simulink model "GoToTest"  (R2015b)
settings: Solver=VariableStepAuto  StartTime=0.0  StopTime=inf  RelTol=1e-3
libraries: aerolibanimutils x1, simulink x1, dspnetwork x1
(part 1 of 2)
settings Model: Creator=Ryuu  LastModifiedBy=Ryuu

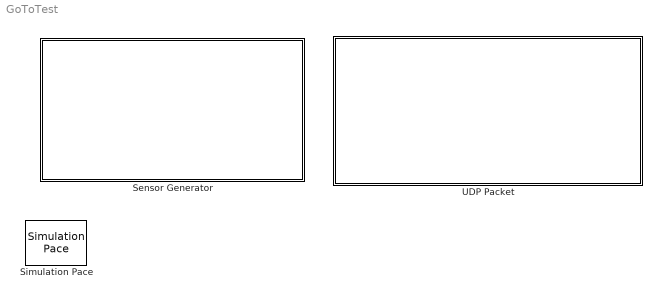
== system GoToTest ==
  "Sensor Generator " : Subsystem
  Simulation Pace : aerolibanimutils/Simulation Pace  SimulationPace=1  SleepMode=MATLAB Thread  OutputPaceError=off  SampleTime=1/30
  UDP Packet : Subsystem

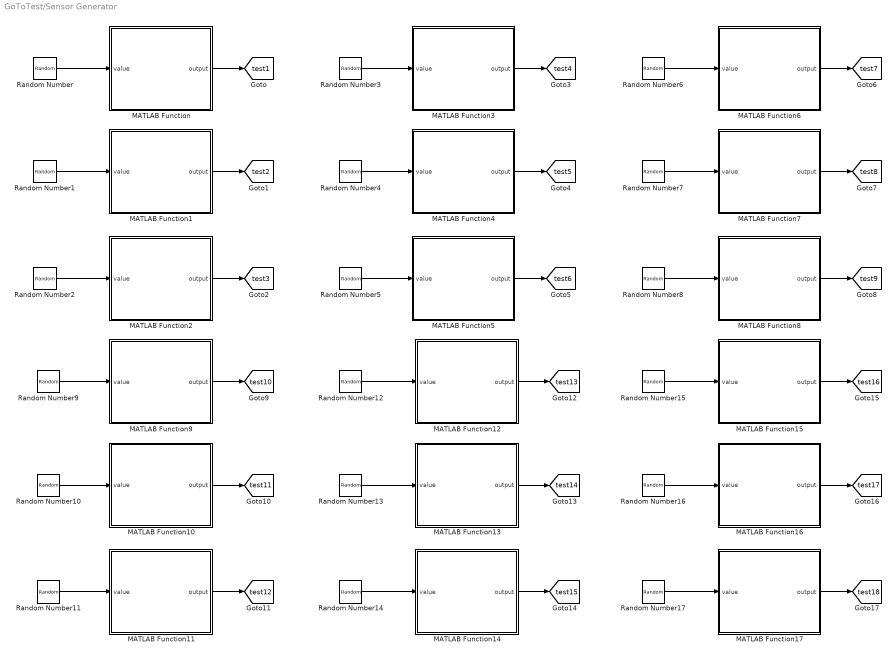
== system GoToTest/Sensor Generator  ==
  MATLAB Function : MATLAB Function  TreatAsAtomicUnit=on
  MATLAB Function1 : MATLAB Function  TreatAsAtomicUnit=on
  MATLAB Function10 : MATLAB Function  TreatAsAtomicUnit=on
  MATLAB Function11 : MATLAB Function  TreatAsAtomicUnit=on
  MATLAB Function12 : MATLAB Function  TreatAsAtomicUnit=on
  MATLAB Function13 : MATLAB Function  TreatAsAtomicUnit=on
  MATLAB Function14 : MATLAB Function  TreatAsAtomicUnit=on
  MATLAB Function15 : MATLAB Function  TreatAsAtomicUnit=on
  MATLAB Function16 : MATLAB Function  TreatAsAtomicUnit=on
  MATLAB Function17 : MATLAB Function  TreatAsAtomicUnit=on
  MATLAB Function2 : MATLAB Function  TreatAsAtomicUnit=on
  MATLAB Function3 : MATLAB Function  TreatAsAtomicUnit=on
  MATLAB Function4 : MATLAB Function  TreatAsAtomicUnit=on
  MATLAB Function5 : MATLAB Function  TreatAsAtomicUnit=on
  MATLAB Function6 : MATLAB Function  TreatAsAtomicUnit=on
  MATLAB Function7 : MATLAB Function  TreatAsAtomicUnit=on
  MATLAB Function8 : MATLAB Function  TreatAsAtomicUnit=on
  MATLAB Function9 : MATLAB Function  TreatAsAtomicUnit=on
  Random Number : RandomNumber  Mean=100  Variance=50  Seed=1  SampleTime=0.02
  Random Number1 : RandomNumber  Mean=100  Variance=50  Seed=2  SampleTime=0.02
  Random Number10 : RandomNumber  Mean=100  Variance=50  Seed=11  SampleTime=0.02
  Random Number11 : RandomNumber  Mean=100  Variance=50  Seed=12  SampleTime=0.02
  Random Number12 : RandomNumber  Mean=100  Variance=50  Seed=13  SampleTime=0.02
  Random Number13 : RandomNumber  Mean=100  Variance=50  Seed=14  SampleTime=0.02
  Random Number14 : RandomNumber  Mean=100  Variance=50  Seed=15  SampleTime=0.02
  Random Number15 : RandomNumber  Mean=100  Variance=50  Seed=16  SampleTime=0.02
  Random Number16 : RandomNumber  Mean=100  Variance=50  Seed=17  SampleTime=0.02
  Random Number17 : RandomNumber  Mean=100  Variance=50  Seed=18  SampleTime=0.02
  Random Number2 : RandomNumber  Mean=100  Variance=50  Seed=3  SampleTime=0.02
  Random Number3 : RandomNumber  Mean=100  Variance=50  Seed=4  SampleTime=0.02
  Random Number4 : RandomNumber  Mean=100  Variance=50  Seed=5  SampleTime=0.02
  Random Number5 : RandomNumber  Mean=100  Variance=50  Seed=6  SampleTime=0.02
  Random Number6 : RandomNumber  Mean=100  Variance=50  Seed=7  SampleTime=0.02
  Random Number7 : RandomNumber  Mean=100  Variance=50  Seed=8  SampleTime=0.02
  Random Number8 : RandomNumber  Mean=100  Variance=50  Seed=9  SampleTime=0.02
  Random Number9 : RandomNumber  Mean=100  Variance=50  Seed=10  SampleTime=0.02
  tag scope: test10=global, test11=global, test12=global, test13=global, test14=global, test15=global, test16=global, test17=global, test18=global, test1=global, test2=global, test3=global, test4=global, test5=global, test6=global, test7=global, test8=global, test9=global
  wires:
  Random Number/1 -> MATLAB Function/1(value)
  MATLAB Function/1(output) -> [test1]
  Random Number1/1 -> MATLAB Function1/1(value)
  MATLAB Function1/1(output) -> [test2]
  Random Number2/1 -> MATLAB Function2/1(value)
  MATLAB Function2/1(output) -> [test3]
  Random Number3/1 -> MATLAB Function3/1(value)
  MATLAB Function3/1(output) -> [test4]
  Random Number4/1 -> MATLAB Function4/1(value)
  MATLAB Function4/1(output) -> [test5]
  Random Number5/1 -> MATLAB Function5/1(value)
  MATLAB Function5/1(output) -> [test6]
  Random Number6/1 -> MATLAB Function6/1(value)
  MATLAB Function6/1(output) -> [test7]
  Random Number7/1 -> MATLAB Function7/1(value)
  MATLAB Function7/1(output) -> [test8]
  Random Number8/1 -> MATLAB Function8/1(value)
  MATLAB Function8/1(output) -> [test9]
  Random Number9/1 -> MATLAB Function9/1(value)
  MATLAB Function9/1(output) -> [test10]
  Random Number10/1 -> MATLAB Function10/1(value)
  MATLAB Function10/1(output) -> [test11]
  Random Number11/1 -> MATLAB Function11/1(value)
  MATLAB Function11/1(output) -> [test12]
  Random Number12/1 -> MATLAB Function12/1(value)
  MATLAB Function12/1(output) -> [test13]
  Random Number13/1 -> MATLAB Function13/1(value)
  MATLAB Function13/1(output) -> [test14]
  Random Number14/1 -> MATLAB Function14/1(value)
  MATLAB Function14/1(output) -> [test15]
  Random Number15/1 -> MATLAB Function15/1(value)
  MATLAB Function15/1(output) -> [test16]
  Random Number16/1 -> MATLAB Function16/1(value)
  MATLAB Function16/1(output) -> [test17]
  Random Number17/1 -> MATLAB Function17/1(value)
  MATLAB Function17/1(output) -> [test18]

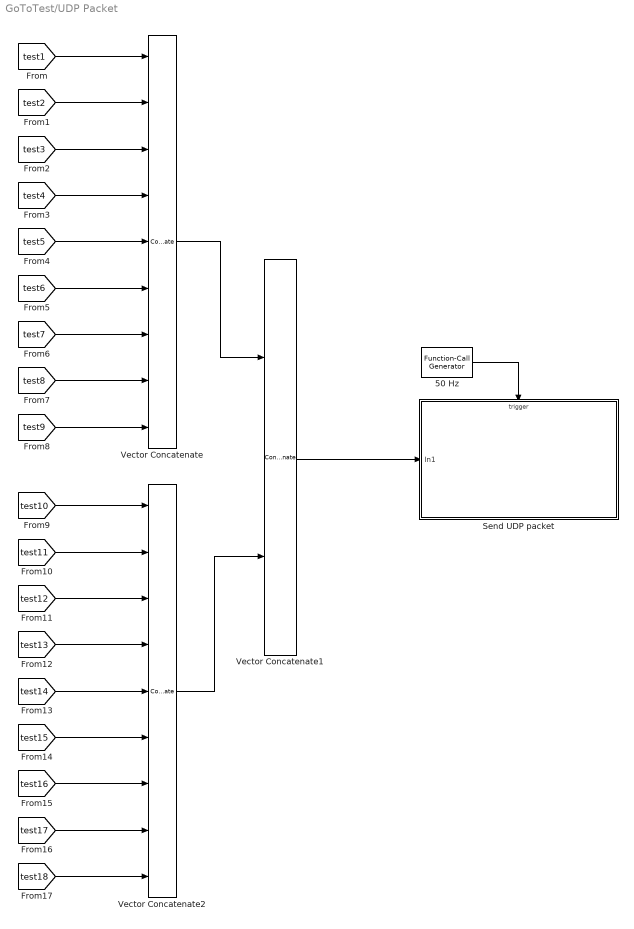
== system GoToTest/UDP Packet ==
  50 Hz : simulink/Ports & Subsystems/Function-Call Generator  sample_time=0.02  numberOfIterations=1
  Send UDP packet : Subsystem
  Vector Concatenate : Concatenate  NumInputs=9
  Vector Concatenate1 : Concatenate
  Vector Concatenate2 : Concatenate  NumInputs=9
  wires:
  [test1] -> Vector Concatenate/1
  50 Hz/1 -> Send UDP packet/Trigger
  Vector Concatenate/1 -> Vector Concatenate1/1
  [test2] -> Vector Concatenate/2
  [test3] -> Vector Concatenate/3
  [test4] -> Vector Concatenate/4
  [test5] -> Vector Concatenate/5
  [test6] -> Vector Concatenate/6
  [test7] -> Vector Concatenate/7
  [test8] -> Vector Concatenate/8
  [test9] -> Vector Concatenate/9
  [test10] -> Vector Concatenate2/1
  [test11] -> Vector Concatenate2/2
  [test12] -> Vector Concatenate2/3
  [test13] -> Vector Concatenate2/4
  [test14] -> Vector Concatenate2/5
  [test15] -> Vector Concatenate2/6
  [test16] -> Vector Concatenate2/7
  [test17] -> Vector Concatenate2/8
  [test18] -> Vector Concatenate2/9
  Vector Concatenate2/1 -> Vector Concatenate1/2
  Vector Concatenate1/1 -> Send UDP packet/1(In1)

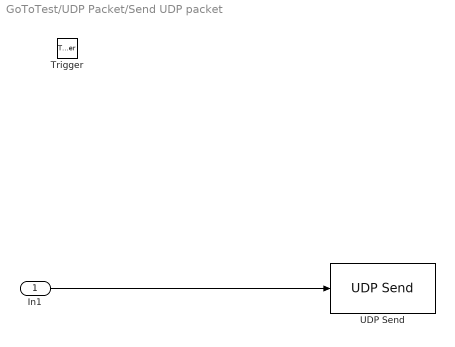
== system GoToTest/UDP Packet/Send UDP packet ==
  In1 : Inport
  Trigger : TriggerPort  TriggerType=function-call  PortDimensions=1
  UDP Send : dspnetwork/UDP Send  remoteURL='192.168.21.1'  remotePort=25000  localURL='0.0.0.0'  localPortSource=Automatically determine  localPort=-1  sampletime=-1  separateLengthPort=0
  wires:
  In1/1 -> UDP Send/1

== matlab function GoToTest/Sensor Generator /MATLAB Function1 ==
  data: value input; output output uint8 size=1000
function output = data_serialize(value)
label = 'Test 2';
type = 'Testsensor 2';
min = 24;
max = 45;

label_ser = sensor_serialize(label);
type_ser = sensor_serialize(type);
value_ser = sensor_serialize(value);
min_ser = sensor_serialize(min);
max_ser = sensor_serialize(max);


V = length(label_ser);
W = length(type_ser);
X = length(value_ser);
Y = length(min_ser);
Z = length(max_ser);

output = [
    label_ser;
    type_ser;
    value_ser;
    min_ser;
    max_ser;
    ];
end


function m = sensor_serialize(v)
    % dispatch according to type
    if isnumeric(v) 
        m = serialize_numeric(v);
    elseif ischar(v)
        m = serialize_string(v);
    elseif islogical(v)
        m = serialize_logical(v);
	else
		error('Unsupported data type');
    end
end

% single scalar
function m = serialize_scalar(v)
    % Data type & data
    m = [class2tag(class(v)); typecast(v,'uint8').'];
end

% char arrays
function m = serialize_string(v)
    if size(v,1) == 1
        % horizontal string: Type, Length, and Data
        m = [uint8(0); typecast(uint32(length(v)),'uint8').'; uint8(v(:))];
    elseif sum(size(v)) == 0
        % '': special encoding
        m = uint8(200);
    else
        % general char array: Tag & Number of dimensions, Dimensions, Data
        m = [uint8(132); ndims(v); typecast(uint32(size(v)),'uint8').'; uint8(v(:))];
    end
end

% logical arrays
function m = serialize_logical(v)
    % Tag & Number of dimensions, Dimensions, Data
    m = [uint8(133); ndims(v); typecast(uint32(size(v)),'uint8').'; uint8(v(:))];
end

% non-complex and non-sparse numerical matrix
function m = serialize_numeric_simple(v)
    % Tag & Number of dimensions, Dimensions, Data
    m = [16+class2tag(class(v)); ndims(v); typecast(uint32(size(v)),'uint8').'; typecast(v(:).','uint8').'];
end

% Numeric Matrix: can be real/complex, sparse/full, scalar
function m = serialize_numeric(v)
    if issparse(v)
        % Data Type & Dimensions
        m = [uint8(130); typecast(uint64(size(v,1)), 'uint8').'; typecast(uint64(size(v,2)), 'uint8').']; % vectorize
        % Index vectors
        [i,j,s] = find(v);        
        % Real/Complex
        if isreal(v)
            m = [m; serialize_numeric_simple(i); serialize_numeric_simple(j); 1; serialize_numeric_simple(s)];
        else
            m = [m; serialize_numeric_simple(i); serialize_numeric_simple(j); 0; serialize_numeric_simple(real(s)); serialize_numeric_simple(imag(s))];
        end
    elseif ~isreal(v)
        % Data type & contents
        m = [uint8(131); serialize_numeric_simple(real(v)); serialize_numeric_simple(imag(v))];
    elseif isscalar(v)
        % Scalar
        m = serialize_scalar(v);
    else
        % Simple matrix
        m = serialize_numeric_simple(v);
    end
end

% *container* class to byte
function b = class2tag(cls)
	switch cls
		case 'string'
            b = uint8(0);
		case 'double'
			b = uint8(1);
		case 'single'
			b = uint8(2);
		case 'int8'
			b = uint8(3);
		case 'uint8'
			b = uint8(4);
		case 'int16'
			b = uint8(5);
		case 'uint16'
			b = uint8(6);
		case 'int32'
			b = uint8(7);
		case 'uint32'
			b = uint8(8);
		case 'int64'
			b = uint8(9);
		case 'uint64'
			b = uint8(10);
		otherwise
			error('Unknown class');
    end
end

== matlab function GoToTest/Sensor Generator /MATLAB Function ==
  data: value input; output output uint8 size=1000
function output = data_serialize(value)
label = 'Test 1';
type = 'Testsensor 1';
min = 24;
max = 45;

label_ser = sensor_serialize(label);
type_ser = sensor_serialize(type);
value_ser = sensor_serialize(value);
min_ser = sensor_serialize(min);
max_ser = sensor_serialize(max);


V = length(label_ser);
W = length(type_ser);
X = length(value_ser);
Y = length(min_ser);
Z = length(max_ser);

output = [
    label_ser;
    type_ser;
    value_ser;
    min_ser;
    max_ser;
    ];
end


function m = sensor_serialize(v)
    % dispatch according to type
    if isnumeric(v) 
        m = serialize_numeric(v);
    elseif ischar(v)
        m = serialize_string(v);
    elseif islogical(v)
        m = serialize_logical(v);
	else
		error('Unsupported data type');
    end
end

% single scalar
function m = serialize_scalar(v)
    % Data type & data
    m = [class2tag(class(v)); typecast(v,'uint8').'];
end

% char arrays
function m = serialize_string(v)
    if size(v,1) == 1
        % horizontal string: Type, Length, and Data
        m = [uint8(0); typecast(uint32(length(v)),'uint8').'; uint8(v(:))];
    elseif sum(size(v)) == 0
        % '': special encoding
        m = uint8(200);
    else
        % general char array: Tag & Number of dimensions, Dimensions, Data
        m = [uint8(132); ndims(v); typecast(uint32(size(v)),'uint8').'; uint8(v(:))];
    end
end

% logical arrays
function m = serialize_logical(v)
    % Tag & Number of dimensions, Dimensions, Data
    m = [uint8(133); ndims(v); typecast(uint32(size(v)),'uint8').'; uint8(v(:))];
end

% non-complex and non-sparse numerical matrix
function m = serialize_numeric_simple(v)
    % Tag & Number of dimensions, Dimensions, Data
    m = [16+class2tag(class(v)); ndims(v); typecast(uint32(size(v)),'uint8').'; typecast(v(:).','uint8').'];
end

% Numeric Matrix: can be real/complex, sparse/full, scalar
function m = serialize_numeric(v)
    if issparse(v)
        % Data Type & Dimensions
        m = [uint8(130); typecast(uint64(size(v,1)), 'uint8').'; typecast(uint64(size(v,2)), 'uint8').']; % vectorize
        % Index vectors
        [i,j,s] = find(v);        
        % Real/Complex
        if isreal(v)
            m = [m; serialize_numeric_simple(i); serialize_numeric_simple(j); 1; serialize_numeric_simple(s)];
        else
            m = [m; serialize_numeric_simple(i); serialize_numeric_simple(j); 0; serialize_numeric_simple(real(s)); serialize_numeric_simple(imag(s))];
        end
    elseif ~isreal(v)
        % Data type & contents
        m = [uint8(131); serialize_numeric_simple(real(v)); serialize_numeric_simple(imag(v))];
    elseif isscalar(v)
        % Scalar
        m = serialize_scalar(v);
    else
        % Simple matrix
        m = serialize_numeric_simple(v);
    end
end

% *container* class to byte
function b = class2tag(cls)
	switch cls
		case 'string'
            b = uint8(0);
		case 'double'
			b = uint8(1);
		case 'single'
			b = uint8(2);
		case 'int8'
			b = uint8(3);
		case 'uint8'
			b = uint8(4);
		case 'int16'
			b = uint8(5);
		case 'uint16'
			b = uint8(6);
		case 'int32'
			b = uint8(7);
		case 'uint32'
			b = uint8(8);
		case 'int64'
			b = uint8(9);
		case 'uint64'
			b = uint8(10);
		otherwise
			error('Unknown class');
    end
end

== matlab function GoToTest/Sensor Generator /MATLAB Function2 ==
  data: value input; output output uint8 size=1000
function output = data_serialize(value)
label = 'Test 3';
type = 'Testsensor 3';
min = 24;
max = 45;

label_ser = sensor_serialize(label);
type_ser = sensor_serialize(type);
value_ser = sensor_serialize(value);
min_ser = sensor_serialize(min);
max_ser = sensor_serialize(max);


V = length(label_ser);
W = length(type_ser);
X = length(value_ser);
Y = length(min_ser);
Z = length(max_ser);

output = [
    label_ser;
    type_ser;
    value_ser;
    min_ser;
    max_ser;
    ];
end


function m = sensor_serialize(v)
    % dispatch according to type
    if isnumeric(v) 
        m = serialize_numeric(v);
    elseif ischar(v)
        m = serialize_string(v);
    elseif islogical(v)
        m = serialize_logical(v);
	else
		error('Unsupported data type');
    end
end

% single scalar
function m = serialize_scalar(v)
    % Data type & data
    m = [class2tag(class(v)); typecast(v,'uint8').'];
end

% char arrays
function m = serialize_string(v)
    if size(v,1) == 1
        % horizontal string: Type, Length, and Data
        m = [uint8(0); typecast(uint32(length(v)),'uint8').'; uint8(v(:))];
    elseif sum(size(v)) == 0
        % '': special encoding
        m = uint8(200);
    else
        % general char array: Tag & Number of dimensions, Dimensions, Data
        m = [uint8(132); ndims(v); typecast(uint32(size(v)),'uint8').'; uint8(v(:))];
    end
end

% logical arrays
function m = serialize_logical(v)
    % Tag & Number of dimensions, Dimensions, Data
    m = [uint8(133); ndims(v); typecast(uint32(size(v)),'uint8').'; uint8(v(:))];
end

% non-complex and non-sparse numerical matrix
function m = serialize_numeric_simple(v)
    % Tag & Number of dimensions, Dimensions, Data
    m = [16+class2tag(class(v)); ndims(v); typecast(uint32(size(v)),'uint8').'; typecast(v(:).','uint8').'];
end

% Numeric Matrix: can be real/complex, sparse/full, scalar
function m = serialize_numeric(v)
    if issparse(v)
        % Data Type & Dimensions
        m = [uint8(130); typecast(uint64(size(v,1)), 'uint8').'; typecast(uint64(size(v,2)), 'uint8').']; % vectorize
        % Index vectors
        [i,j,s] = find(v);        
        % Real/Complex
        if isreal(v)
            m = [m; serialize_numeric_simple(i); serialize_numeric_simple(j); 1; serialize_numeric_simple(s)];
        else
            m = [m; serialize_numeric_simple(i); serialize_numeric_simple(j); 0; serialize_numeric_simple(real(s)); serialize_numeric_simple(imag(s))];
        end
    elseif ~isreal(v)
        % Data type & contents
        m = [uint8(131); serialize_numeric_simple(real(v)); serialize_numeric_simple(imag(v))];
    elseif isscalar(v)
        % Scalar
        m = serialize_scalar(v);
    else
        % Simple matrix
        m = serialize_numeric_simple(v);
    end
end

% *container* class to byte
function b = class2tag(cls)
	switch cls
		case 'string'
            b = uint8(0);
		case 'double'
			b = uint8(1);
		case 'single'
			b = uint8(2);
		case 'int8'
			b = uint8(3);
		case 'uint8'
			b = uint8(4);
		case 'int16'
			b = uint8(5);
		case 'uint16'
			b = uint8(6);
		case 'int32'
			b = uint8(7);
		case 'uint32'
			b = uint8(8);
		case 'int64'
			b = uint8(9);
		case 'uint64'
			b = uint8(10);
		otherwise
			error('Unknown class');
    end
end

== matlab function GoToTest/Sensor Generator /MATLAB Function3 ==
  data: value input; output output uint8 size=1000
function output = data_serialize(value)
label = 'Test 4';
type = 'Testsensor 4';
min = 24;
max = 45;

label_ser = sensor_serialize(label);
type_ser = sensor_serialize(type);
value_ser = sensor_serialize(value);
min_ser = sensor_serialize(min);
max_ser = sensor_serialize(max);


V = length(label_ser);
W = length(type_ser);
X = length(value_ser);
Y = length(min_ser);
Z = length(max_ser);

output = [
    label_ser;
    type_ser;
    value_ser;
    min_ser;
    max_ser;
    ];
end


function m = sensor_serialize(v)
    % dispatch according to type
    if isnumeric(v) 
        m = serialize_numeric(v);
    elseif ischar(v)
        m = serialize_string(v);
    elseif islogical(v)
        m = serialize_logical(v);
	else
		error('Unsupported data type');
    end
end

% single scalar
function m = serialize_scalar(v)
    % Data type & data
    m = [class2tag(class(v)); typecast(v,'uint8').'];
end

% char arrays
function m = serialize_string(v)
    if size(v,1) == 1
        % horizontal string: Type, Length, and Data
        m = [uint8(0); typecast(uint32(length(v)),'uint8').'; uint8(v(:))];
    elseif sum(size(v)) == 0
        % '': special encoding
        m = uint8(200);
    else
        % general char array: Tag & Number of dimensions, Dimensions, Data
        m = [uint8(132); ndims(v); typecast(uint32(size(v)),'uint8').'; uint8(v(:))];
    end
end

% logical arrays
function m = serialize_logical(v)
    % Tag & Number of dimensions, Dimensions, Data
    m = [uint8(133); ndims(v); typecast(uint32(size(v)),'uint8').'; uint8(v(:))];
end

% non-complex and non-sparse numerical matrix
function m = serialize_numeric_simple(v)
    % Tag & Number of dimensions, Dimensions, Data
    m = [16+class2tag(class(v)); ndims(v); typecast(uint32(size(v)),'uint8').'; typecast(v(:).','uint8').'];
end

% Numeric Matrix: can be real/complex, sparse/full, scalar
function m = serialize_numeric(v)
    if issparse(v)
        % Data Type & Dimensions
        m = [uint8(130); typecast(uint64(size(v,1)), 'uint8').'; typecast(uint64(size(v,2)), 'uint8').']; % vectorize
        % Index vectors
        [i,j,s] = find(v);        
        % Real/Complex
        if isreal(v)
            m = [m; serialize_numeric_simple(i); serialize_numeric_simple(j); 1; serialize_numeric_simple(s)];
        else
            m = [m; serialize_numeric_simple(i); serialize_numeric_simple(j); 0; serialize_numeric_simple(real(s)); serialize_numeric_simple(imag(s))];
        end
    elseif ~isreal(v)
        % Data type & contents
        m = [uint8(131); serialize_numeric_simple(real(v)); serialize_numeric_simple(imag(v))];
    elseif isscalar(v)
        % Scalar
        m = serialize_scalar(v);
    else
        % Simple matrix
        m = serialize_numeric_simple(v);
    end
end

% *container* class to byte
function b = class2tag(cls)
	switch cls
		case 'string'
            b = uint8(0);
		case 'double'
			b = uint8(1);
		case 'single'
			b = uint8(2);
		case 'int8'
			b = uint8(3);
		case 'uint8'
			b = uint8(4);
		case 'int16'
			b = uint8(5);
		case 'uint16'
			b = uint8(6);
		case 'int32'
			b = uint8(7);
		case 'uint32'
			b = uint8(8);
		case 'int64'
			b = uint8(9);
		case 'uint64'
			b = uint8(10);
		otherwise
			error('Unknown class');
    end
end

== matlab function GoToTest/Sensor Generator /MATLAB Function4 ==
  data: value input; output output uint8 size=1000
function output = data_serialize(value)
label = 'Test 5';
type = 'Testsensor 5';
min = 24;
max = 45;

label_ser = sensor_serialize(label);
type_ser = sensor_serialize(type);
value_ser = sensor_serialize(value);
min_ser = sensor_serialize(min);
max_ser = sensor_serialize(max);


V = length(label_ser);
W = length(type_ser);
X = length(value_ser);
Y = length(min_ser);
Z = length(max_ser);

output = [
    label_ser;
    type_ser;
    value_ser;
    min_ser;
    max_ser;
    ];
end


function m = sensor_serialize(v)
    % dispatch according to type
    if isnumeric(v) 
        m = serialize_numeric(v);
    elseif ischar(v)
        m = serialize_string(v);
    elseif islogical(v)
        m = serialize_logical(v);
	else
		error('Unsupported data type');
    end
end

% single scalar
function m = serialize_scalar(v)
    % Data type & data
    m = [class2tag(class(v)); typecast(v,'uint8').'];
end

% char arrays
function m = serialize_string(v)
    if size(v,1) == 1
        % horizontal string: Type, Length, and Data
        m = [uint8(0); typecast(uint32(length(v)),'uint8').'; uint8(v(:))];
    elseif sum(size(v)) == 0
        % '': special encoding
        m = uint8(200);
    else
        % general char array: Tag & Number of dimensions, Dimensions, Data
        m = [uint8(132); ndims(v); typecast(uint32(size(v)),'uint8').'; uint8(v(:))];
    end
end

% logical arrays
function m = serialize_logical(v)
    % Tag & Number of dimensions, Dimensions, Data
    m = [uint8(133); ndims(v); typecast(uint32(size(v)),'uint8').'; uint8(v(:))];
end

% non-complex and non-sparse numerical matrix
function m = serialize_numeric_simple(v)
    % Tag & Number of dimensions, Dimensions, Data
    m = [16+class2tag(class(v)); ndims(v); typecast(uint32(size(v)),'uint8').'; typecast(v(:).','uint8').'];
end

% Numeric Matrix: can be real/complex, sparse/full, scalar
function m = serialize_numeric(v)
    if issparse(v)
        % Data Type & Dimensions
        m = [uint8(130); typecast(uint64(size(v,1)), 'uint8').'; typecast(uint64(size(v,2)), 'uint8').']; % vectorize
        % Index vectors
        [i,j,s] = find(v);        
        % Real/Complex
        if isreal(v)
            m = [m; serialize_numeric_simple(i); serialize_numeric_simple(j); 1; serialize_numeric_simple(s)];
        else
            m = [m; serialize_numeric_simple(i); serialize_numeric_simple(j); 0; serialize_numeric_simple(real(s)); serialize_numeric_simple(imag(s))];
        end
    elseif ~isreal(v)
        % Data type & contents
        m = [uint8(131); serialize_numeric_simple(real(v)); serialize_numeric_simple(imag(v))];
    elseif isscalar(v)
        % Scalar
        m = serialize_scalar(v);
    else
        % Simple matrix
        m = serialize_numeric_simple(v);
    end
end

% *container* class to byte
function b = class2tag(cls)
	switch cls
		case 'string'
            b = uint8(0);
		case 'double'
			b = uint8(1);
		case 'single'
			b = uint8(2);
		case 'int8'
			b = uint8(3);
		case 'uint8'
			b = uint8(4);
		case 'int16'
			b = uint8(5);
		case 'uint16'
			b = uint8(6);
		case 'int32'
			b = uint8(7);
		case 'uint32'
			b = uint8(8);
		case 'int64'
			b = uint8(9);
		case 'uint64'
			b = uint8(10);
		otherwise
			error('Unknown class');
    end
end

== matlab function GoToTest/Sensor Generator /MATLAB Function5 ==
  data: value input; output output uint8 size=1000
function output = data_serialize(value)
label = 'Test 6';
type = 'Testsensor 6';
min = 24;
max = 45;

label_ser = sensor_serialize(label);
type_ser = sensor_serialize(type);
value_ser = sensor_serialize(value);
min_ser = sensor_serialize(min);
max_ser = sensor_serialize(max);


V = length(label_ser);
W = length(type_ser);
X = length(value_ser);
Y = length(min_ser);
Z = length(max_ser);

output = [
    label_ser;
    type_ser;
    value_ser;
    min_ser;
    max_ser;
    ];
end


function m = sensor_serialize(v)
    % dispatch according to type
    if isnumeric(v) 
        m = serialize_numeric(v);
    elseif ischar(v)
        m = serialize_string(v);
    elseif islogical(v)
        m = serialize_logical(v);
	else
		error('Unsupported data type');
    end
end

% single scalar
function m = serialize_scalar(v)
    % Data type & data
    m = [class2tag(class(v)); typecast(v,'uint8').'];
end

% char arrays
function m = serialize_string(v)
    if size(v,1) == 1
        % horizontal string: Type, Length, and Data
        m = [uint8(0); typecast(uint32(length(v)),'uint8').'; uint8(v(:))];
    elseif sum(size(v)) == 0
        % '': special encoding
        m = uint8(200);
    else
        % general char array: Tag & Number of dimensions, Dimensions, Data
        m = [uint8(132); ndims(v); typecast(uint32(size(v)),'uint8').'; uint8(v(:))];
    end
end

% logical arrays
function m = serialize_logical(v)
    % Tag & Number of dimensions, Dimensions, Data
    m = [uint8(133); ndims(v); typecast(uint32(size(v)),'uint8').'; uint8(v(:))];
end

% non-complex and non-sparse numerical matrix
function m = serialize_numeric_simple(v)
    % Tag & Number of dimensions, Dimensions, Data
    m = [16+class2tag(class(v)); ndims(v); typecast(uint32(size(v)),'uint8').'; typecast(v(:).','uint8').'];
end

% Numeric Matrix: can be real/complex, sparse/full, scalar
function m = serialize_numeric(v)
    if issparse(v)
        % Data Type & Dimensions
        m = [uint8(130); typecast(uint64(size(v,1)), 'uint8').'; typecast(uint64(size(v,2)), 'uint8').']; % vectorize
        % Index vectors
        [i,j,s] = find(v);        
        % Real/Complex
        if isreal(v)
            m = [m; serialize_numeric_simple(i); serialize_numeric_simple(j); 1; serialize_numeric_simple(s)];
        else
            m = [m; serialize_numeric_simple(i); serialize_numeric_simple(j); 0; serialize_numeric_simple(real(s)); serialize_numeric_simple(imag(s))];
        end
    elseif ~isreal(v)
        % Data type & contents
        m = [uint8(131); serialize_numeric_simple(real(v)); serialize_numeric_simple(imag(v))];
    elseif isscalar(v)
        % Scalar
        m = serialize_scalar(v);
    else
        % Simple matrix
        m = serialize_numeric_simple(v);
    end
end

% *container* class to byte
function b = class2tag(cls)
	switch cls
		case 'string'
            b = uint8(0);
		case 'double'
			b = uint8(1);
		case 'single'
			b = uint8(2);
		case 'int8'
			b = uint8(3);
		case 'uint8'
			b = uint8(4);
		case 'int16'
			b = uint8(5);
		case 'uint16'
			b = uint8(6);
		case 'int32'
			b = uint8(7);
		case 'uint32'
			b = uint8(8);
		case 'int64'
			b = uint8(9);
		case 'uint64'
			b = uint8(10);
		otherwise
			error('Unknown class');
    end
end

== matlab function GoToTest/Sensor Generator /MATLAB Function6 ==
  data: value input; output output uint8 size=1000
function output = data_serialize(value)
label = 'Test 7';
type = 'Testsensor 7';
min = 24;
max = 45;

label_ser = sensor_serialize(label);
type_ser = sensor_serialize(type);
value_ser = sensor_serialize(value);
min_ser = sensor_serialize(min);
max_ser = sensor_serialize(max);


V = length(label_ser);
W = length(type_ser);
X = length(value_ser);
Y = length(min_ser);
Z = length(max_ser);

output = [
    label_ser;
    type_ser;
    value_ser;
    min_ser;
    max_ser;
    ];
end


function m = sensor_serialize(v)
    % dispatch according to type
    if isnumeric(v) 
        m = serialize_numeric(v);
    elseif ischar(v)
        m = serialize_string(v);
    elseif islogical(v)
        m = serialize_logical(v);
	else
		error('Unsupported data type');
    end
end

% single scalar
function m = serialize_scalar(v)
    % Data type & data
    m = [class2tag(class(v)); typecast(v,'uint8').'];
end

% char arrays
function m = serialize_string(v)
    if size(v,1) == 1
        % horizontal string: Type, Length, and Data
        m = [uint8(0); typecast(uint32(length(v)),'uint8').'; uint8(v(:))];
    elseif sum(size(v)) == 0
        % '': special encoding
        m = uint8(200);
    else
        % general char array: Tag & Number of dimensions, Dimensions, Data
        m = [uint8(132); ndims(v); typecast(uint32(size(v)),'uint8').'; uint8(v(:))];
    end
end

% logical arrays
function m = serialize_logical(v)
    % Tag & Number of dimensions, Dimensions, Data
    m = [uint8(133); ndims(v); typecast(uint32(size(v)),'uint8').'; uint8(v(:))];
end

% non-complex and non-sparse numerical matrix
function m = serialize_numeric_simple(v)
    % Tag & Number of dimensions, Dimensions, Data
    m = [16+class2tag(class(v)); ndims(v); typecast(uint32(size(v)),'uint8').'; typecast(v(:).','uint8').'];
end

% Numeric Matrix: can be real/complex, sparse/full, scalar
function m = serialize_numeric(v)
    if issparse(v)
        % Data Type & Dimensions
        m = [uint8(130); typecast(uint64(size(v,1)), 'uint8').'; typecast(uint64(size(v,2)), 'uint8').']; % vectorize
        % Index vectors
        [i,j,s] = find(v);        
        % Real/Complex
        if isreal(v)
            m = [m; serialize_numeric_simple(i); serialize_numeric_simple(j); 1; serialize_numeric_simple(s)];
        else
            m = [m; serialize_numeric_simple(i); serialize_numeric_simple(j); 0; serialize_numeric_simple(real(s)); serialize_numeric_simple(imag(s))];
        end
    elseif ~isreal(v)
        % Data type & contents
        m = [uint8(131); serialize_numeric_simple(real(v)); serialize_numeric_simple(imag(v))];
    elseif isscalar(v)
        % Scalar
        m = serialize_scalar(v);
    else
        % Simple matrix
        m = serialize_numeric_simple(v);
    end
end

% *container* class to byte
function b = class2tag(cls)
	switch cls
		case 'string'
            b = uint8(0);
		case 'double'
			b = uint8(1);
		case 'single'
			b = uint8(2);
		case 'int8'
			b = uint8(3);
		case 'uint8'
			b = uint8(4);
		case 'int16'
			b = uint8(5);
		case 'uint16'
			b = uint8(6);
		case 'int32'
			b = uint8(7);
		case 'uint32'
			b = uint8(8);
		case 'int64'
			b = uint8(9);
		case 'uint64'
			b = uint8(10);
		otherwise
			error('Unknown class');
    end
end

== matlab function GoToTest/Sensor Generator /MATLAB Function7 ==
  data: value input; output output uint8 size=1000
function output = data_serialize(value)
label = 'Test 8';
type = 'Testsensor 8';
min = 24;
max = 45;

label_ser = sensor_serialize(label);
type_ser = sensor_serialize(type);
value_ser = sensor_serialize(value);
min_ser = sensor_serialize(min);
max_ser = sensor_serialize(max);


V = length(label_ser);
W = length(type_ser);
X = length(value_ser);
Y = length(min_ser);
Z = length(max_ser);

output = [
    label_ser;
    type_ser;
    value_ser;
    min_ser;
    max_ser;
    ];
end


function m = sensor_serialize(v)
    % dispatch according to type
    if isnumeric(v) 
        m = serialize_numeric(v);
    elseif ischar(v)
        m = serialize_string(v);
    elseif islogical(v)
        m = serialize_logical(v);
	else
		error('Unsupported data type');
    end
end

% single scalar
function m = serialize_scalar(v)
    % Data type & data
    m = [class2tag(class(v)); typecast(v,'uint8').'];
end

% char arrays
function m = serialize_string(v)
    if size(v,1) == 1
        % horizontal string: Type, Length, and Data
        m = [uint8(0); typecast(uint32(length(v)),'uint8').'; uint8(v(:))];
    elseif sum(size(v)) == 0
        % '': special encoding
        m = uint8(200);
    else
        % general char array: Tag & Number of dimensions, Dimensions, Data
        m = [uint8(132); ndims(v); typecast(uint32(size(v)),'uint8').'; uint8(v(:))];
    end
end

% logical arrays
function m = serialize_logical(v)
    % Tag & Number of dimensions, Dimensions, Data
    m = [uint8(133); ndims(v); typecast(uint32(size(v)),'uint8').'; uint8(v(:))];
end

% non-complex and non-sparse numerical matrix
function m = serialize_numeric_simple(v)
    % Tag & Number of dimensions, Dimensions, Data
    m = [16+class2tag(class(v)); ndims(v); typecast(uint32(size(v)),'uint8').'; typecast(v(:).','uint8').'];
end

% Numeric Matrix: can be real/complex, sparse/full, scalar
function m = serialize_numeric(v)
    if issparse(v)
        % Data Type & Dimensions
        m = [uint8(130); typecast(uint64(size(v,1)), 'uint8').'; typecast(uint64(size(v,2)), 'uint8').']; % vectorize
        % Index vectors
        [i,j,s] = find(v);        
        % Real/Complex
        if isreal(v)
            m = [m; serialize_numeric_simple(i); serialize_numeric_simple(j); 1; serialize_numeric_simple(s)];
        else
            m = [m; serialize_numeric_simple(i); serialize_numeric_simple(j); 0; serialize_numeric_simple(real(s)); serialize_numeric_simple(imag(s))];
        end
    elseif ~isreal(v)
        % Data type & contents
        m = [uint8(131); serialize_numeric_simple(real(v)); serialize_numeric_simple(imag(v))];
    elseif isscalar(v)
        % Scalar
        m = serialize_scalar(v);
    else
        % Simple matrix
        m = serialize_numeric_simple(v);
    end
end

% *container* class to byte
function b = class2tag(cls)
	switch cls
		case 'string'
            b = uint8(0);
		case 'double'
			b = uint8(1);
		case 'single'
			b = uint8(2);
		case 'int8'
			b = uint8(3);
		case 'uint8'
			b = uint8(4);
		case 'int16'
			b = uint8(5);
		case 'uint16'
			b = uint8(6);
		case 'int32'
			b = uint8(7);
		case 'uint32'
			b = uint8(8);
		case 'int64'
			b = uint8(9);
		case 'uint64'
			b = uint8(10);
		otherwise
			error('Unknown class');
    end
end

== matlab function GoToTest/Sensor Generator /MATLAB Function8 ==
  data: value input; output output uint8 size=1000
function output = data_serialize(value)
label = 'Test 9';
type = 'Testsensor 9';
min = 24;
max = 45;

label_ser = sensor_serialize(label);
type_ser = sensor_serialize(type);
value_ser = sensor_serialize(value);
min_ser = sensor_serialize(min);
max_ser = sensor_serialize(max);


V = length(label_ser);
W = length(type_ser);
X = length(value_ser);
Y = length(min_ser);
Z = length(max_ser);

output = [
    label_ser;
    type_ser;
    value_ser;
    min_ser;
    max_ser;
    ];
end


function m = sensor_serialize(v)
    % dispatch according to type
    if isnumeric(v) 
        m = serialize_numeric(v);
    elseif ischar(v)
        m = serialize_string(v);
    elseif islogical(v)
        m = serialize_logical(v);
	else
		error('Unsupported data type');
    end
end

% single scalar
function m = serialize_scalar(v)
    % Data type & data
    m = [class2tag(class(v)); typecast(v,'uint8').'];
end

% char arrays
function m = serialize_string(v)
    if size(v,1) == 1
        % horizontal string: Type, Length, and Data
        m = [uint8(0); typecast(uint32(length(v)),'uint8').'; uint8(v(:))];
    elseif sum(size(v)) == 0
        % '': special encoding
        m = uint8(200);
    else
        % general char array: Tag & Number of dimensions, Dimensions, Data
        m = [uint8(132); ndims(v); typecast(uint32(size(v)),'uint8').'; uint8(v(:))];
    end
end

% logical arrays
function m = serialize_logical(v)
    % Tag & Number of dimensions, Dimensions, Data
    m = [uint8(133); ndims(v); typecast(uint32(size(v)),'uint8').'; uint8(v(:))];
end

% non-complex and non-sparse numerical matrix
function m = serialize_numeric_simple(v)
    % Tag & Number of dimensions, Dimensions, Data
    m = [16+class2tag(class(v)); ndims(v); typecast(uint32(size(v)),'uint8').'; typecast(v(:).','uint8').'];
end

% Numeric Matrix: can be real/complex, sparse/full, scalar
function m = serialize_numeric(v)
    if issparse(v)
        % Data Type & Dimensions
        m = [uint8(130); typecast(uint64(size(v,1)), 'uint8').'; typecast(uint64(size(v,2)), 'uint8').']; % vectorize
        % Index vectors
        [i,j,s] = find(v);        
        % Real/Complex
        if isreal(v)
            m = [m; serialize_numeric_simple(i); serialize_numeric_simple(j); 1; serialize_numeric_simple(s)];
        else
            m = [m; serialize_numeric_simple(i); serialize_numeric_simple(j); 0; serialize_numeric_simple(real(s)); serialize_numeric_simple(imag(s))];
        end
    elseif ~isreal(v)
        % Data type & contents
        m = [uint8(131); serialize_numeric_simple(real(v)); serialize_numeric_simple(imag(v))];
    elseif isscalar(v)
        % Scalar
        m = serialize_scalar(v);
    else
        % Simple matrix
        m = serialize_numeric_simple(v);
    end
end

% *container* class to byte
function b = class2tag(cls)
	switch cls
		case 'string'
            b = uint8(0);
		case 'double'
			b = uint8(1);
		case 'single'
			b = uint8(2);
		case 'int8'
			b = uint8(3);
		case 'uint8'
			b = uint8(4);
		case 'int16'
			b = uint8(5);
		case 'uint16'
			b = uint8(6);
		case 'int32'
			b = uint8(7);
		case 'uint32'
			b = uint8(8);
		case 'int64'
			b = uint8(9);
		case 'uint64'
			b = uint8(10);
		otherwise
			error('Unknown class');
    end
end

== matlab function GoToTest/Sensor Generator /MATLAB Function10 ==
  data: value input; output output uint8 size=1000
function output = data_serialize(value)
label = 'Test 11';
type = 'Testsensor 11';
min = 24;
max = 45;

label_ser = sensor_serialize(label);
type_ser = sensor_serialize(type);
value_ser = sensor_serialize(value);
min_ser = sensor_serialize(min);
max_ser = sensor_serialize(max);


V = length(label_ser);
W = length(type_ser);
X = length(value_ser);
Y = length(min_ser);
Z = length(max_ser);

output = [
    label_ser;
    type_ser;
    value_ser;
    min_ser;
    max_ser;
    ];
end


function m = sensor_serialize(v)
    % dispatch according to type
    if isnumeric(v) 
        m = serialize_numeric(v);
    elseif ischar(v)
        m = serialize_string(v);
    elseif islogical(v)
        m = serialize_logical(v);
	else
		error('Unsupported data type');
    end
end

% single scalar
function m = serialize_scalar(v)
    % Data type & data
    m = [class2tag(class(v)); typecast(v,'uint8').'];
end

% char arrays
function m = serialize_string(v)
    if size(v,1) == 1
        % horizontal string: Type, Length, and Data
        m = [uint8(0); typecast(uint32(length(v)),'uint8').'; uint8(v(:))];
    elseif sum(size(v)) == 0
        % '': special encoding
        m = uint8(200);
    else
        % general char array: Tag & Number of dimensions, Dimensions, Data
        m = [uint8(132); ndims(v); typecast(uint32(size(v)),'uint8').'; uint8(v(:))];
    end
end

% logical arrays
function m = serialize_logical(v)
    % Tag & Number of dimensions, Dimensions, Data
    m = [uint8(133); ndims(v); typecast(uint32(size(v)),'uint8').'; uint8(v(:))];
end

% non-complex and non-sparse numerical matrix
function m = serialize_numeric_simple(v)
    % Tag & Number of dimensions, Dimensions, Data
    m = [16+class2tag(class(v)); ndims(v); typecast(uint32(size(v)),'uint8').'; typecast(v(:).','uint8').'];
end

% Numeric Matrix: can be real/complex, sparse/full, scalar
function m = serialize_numeric(v)
    if issparse(v)
        % Data Type & Dimensions
        m = [uint8(130); typecast(uint64(size(v,1)), 'uint8').'; typecast(uint64(size(v,2)), 'uint8').']; % vectorize
        % Index vectors
        [i,j,s] = find(v);        
        % Real/Complex
        if isreal(v)
            m = [m; serialize_numeric_simple(i); serialize_numeric_simple(j); 1; serialize_numeric_simple(s)];
        else
            m = [m; serialize_numeric_simple(i); serialize_numeric_simple(j); 0; serialize_numeric_simple(real(s)); serialize_numeric_simple(imag(s))];
        end
    elseif ~isreal(v)
        % Data type & contents
        m = [uint8(131); serialize_numeric_simple(real(v)); serialize_numeric_simple(imag(v))];
    elseif isscalar(v)
        % Scalar
        m = serialize_scalar(v);
    else
        % Simple matrix
        m = serialize_numeric_simple(v);
    end
end

% *container* class to byte
function b = class2tag(cls)
	switch cls
		case 'string'
            b = uint8(0);
		case 'double'
			b = uint8(1);
		case 'single'
			b = uint8(2);
		case 'int8'
			b = uint8(3);
		case 'uint8'
			b = uint8(4);
		case 'int16'
			b = uint8(5);
		case 'uint16'
			b = uint8(6);
		case 'int32'
			b = uint8(7);
		case 'uint32'
			b = uint8(8);
		case 'int64'
			b = uint8(9);
		case 'uint64'
			b = uint8(10);
		otherwise
			error('Unknown class');
    end
end

== matlab function GoToTest/Sensor Generator /MATLAB Function11 ==
  data: value input; output output uint8 size=1000
function output = data_serialize(value)
label = 'Test 12';
type = 'Testsensor 12';
min = 24;
max = 45;

label_ser = sensor_serialize(label);
type_ser = sensor_serialize(type);
value_ser = sensor_serialize(value);
min_ser = sensor_serialize(min);
max_ser = sensor_serialize(max);


V = length(label_ser);
W = length(type_ser);
X = length(value_ser);
Y = length(min_ser);
Z = length(max_ser);

output = [
    label_ser;
    type_ser;
    value_ser;
    min_ser;
    max_ser;
    ];
end


function m = sensor_serialize(v)
    % dispatch according to type
    if isnumeric(v) 
        m = serialize_numeric(v);
    elseif ischar(v)
        m = serialize_string(v);
    elseif islogical(v)
        m = serialize_logical(v);
	else
		error('Unsupported data type');
    end
end

% single scalar
function m = serialize_scalar(v)
    % Data type & data
    m = [class2tag(class(v)); typecast(v,'uint8').'];
end

% char arrays
function m = serialize_string(v)
    if size(v,1) == 1
        % horizontal string: Type, Length, and Data
        m = [uint8(0); typecast(uint32(length(v)),'uint8').'; uint8(v(:))];
    elseif sum(size(v)) == 0
        % '': special encoding
        m = uint8(200);
    else
        % general char array: Tag & Number of dimensions, Dimensions, Data
        m = [uint8(132); ndims(v); typecast(uint32(size(v)),'uint8').'; uint8(v(:))];
    end
end

% logical arrays
function m = serialize_logical(v)
    % Tag & Number of dimensions, Dimensions, Data
    m = [uint8(133); ndims(v); typecast(uint32(size(v)),'uint8').'; uint8(v(:))];
end

% non-complex and non-sparse numerical matrix
function m = serialize_numeric_simple(v)
    % Tag & Number of dimensions, Dimensions, Data
    m = [16+class2tag(class(v)); ndims(v); typecast(uint32(size(v)),'uint8').'; typecast(v(:).','uint8').'];
end

% Numeric Matrix: can be real/complex, sparse/full, scalar
function m = serialize_numeric(v)
    if issparse(v)
        % Data Type & Dimensions
        m = [uint8(130); typecast(uint64(size(v,1)), 'uint8').'; typecast(uint64(size(v,2)), 'uint8').']; % vectorize
        % Index vectors
        [i,j,s] = find(v);        
        % Real/Complex
        if isreal(v)
            m = [m; serialize_numeric_simple(i); serialize_numeric_simple(j); 1; serialize_numeric_simple(s)];
        else
            m = [m; serialize_numeric_simple(i); serialize_numeric_simple(j); 0; serialize_numeric_simple(real(s)); serialize_numeric_simple(imag(s))];
        end
    elseif ~isreal(v)
        % Data type & contents
        m = [uint8(131); serialize_numeric_simple(real(v)); serialize_numeric_simple(imag(v))];
    elseif isscalar(v)
        % Scalar
        m = serialize_scalar(v);
    else
        % Simple matrix
        m = serialize_numeric_simple(v);
    end
end

% *container* class to byte
function b = class2tag(cls)
	switch cls
		case 'string'
            b = uint8(0);
		case 'double'
			b = uint8(1);
		case 'single'
			b = uint8(2);
		case 'int8'
			b = uint8(3);
		case 'uint8'
			b = uint8(4);
		case 'int16'
			b = uint8(5);
		case 'uint16'
			b = uint8(6);
		case 'int32'
			b = uint8(7);
		case 'uint32'
			b = uint8(8);
		case 'int64'
			b = uint8(9);
		case 'uint64'
			b = uint8(10);
		otherwise
			error('Unknown class');
    end
end

== matlab function GoToTest/Sensor Generator /MATLAB Function12 ==
  data: value input; output output uint8 size=1000
function output = data_serialize(value)
label = 'Test 13';
type = 'Testsensor 13';
min = 24;
max = 45;

label_ser = sensor_serialize(label);
type_ser = sensor_serialize(type);
value_ser = sensor_serialize(value);
min_ser = sensor_serialize(min);
max_ser = sensor_serialize(max);


V = length(label_ser);
W = length(type_ser);
X = length(value_ser);
Y = length(min_ser);
Z = length(max_ser);

output = [
    label_ser;
    type_ser;
    value_ser;
    min_ser;
    max_ser;
    ];
end


function m = sensor_serialize(v)
    % dispatch according to type
    if isnumeric(v) 
        m = serialize_numeric(v);
    elseif ischar(v)
        m = serialize_string(v);
    elseif islogical(v)
        m = serialize_logical(v);
	else
		error('Unsupported data type');
    end
end

% single scalar
function m = serialize_scalar(v)
    % Data type & data
    m = [class2tag(class(v)); typecast(v,'uint8').'];
end

% char arrays
function m = serialize_string(v)
    if size(v,1) == 1
        % horizontal string: Type, Length, and Data
        m = [uint8(0); typecast(uint32(length(v)),'uint8').'; uint8(v(:))];
    elseif sum(size(v)) == 0
        % '': special encoding
        m = uint8(200);
    else
        % general char array: Tag & Number of dimensions, Dimensions, Data
        m = [uint8(132); ndims(v); typecast(uint32(size(v)),'uint8').'; uint8(v(:))];
    end
end

% logical arrays
function m = serialize_logical(v)
    % Tag & Number of dimensions, Dimensions, Data
    m = [uint8(133); ndims(v); typecast(uint32(size(v)),'uint8').'; uint8(v(:))];
end

% non-complex and non-sparse numerical matrix
function m = serialize_numeric_simple(v)
    % Tag & Number of dimensions, Dimensions, Data
    m = [16+class2tag(class(v)); ndims(v); typecast(uint32(size(v)),'uint8').'; typecast(v(:).','uint8').'];
end

% Numeric Matrix: can be real/complex, sparse/full, scalar
function m = serialize_numeric(v)
    if issparse(v)
        % Data Type & Dimensions
        m = [uint8(130); typecast(uint64(size(v,1)), 'uint8').'; typecast(uint64(size(v,2)), 'uint8').']; % vectorize
        % Index vectors
        [i,j,s] = find(v);        
        % Real/Complex
        if isreal(v)
            m = [m; serialize_numeric_simple(i); serialize_numeric_simple(j); 1; serialize_numeric_simple(s)];
        else
            m = [m; serialize_numeric_simple(i); serialize_numeric_simple(j); 0; serialize_numeric_simple(real(s)); serialize_numeric_simple(imag(s))];
        end
    elseif ~isreal(v)
        % Data type & contents
        m = [uint8(131); serialize_numeric_simple(real(v)); serialize_numeric_simple(imag(v))];
    elseif isscalar(v)
        % Scalar
        m = serialize_scalar(v);
    else
        % Simple matrix
        m = serialize_numeric_simple(v);
    end
end

% *container* class to byte
function b = class2tag(cls)
	switch cls
		case 'string'
            b = uint8(0);
		case 'double'
			b = uint8(1);
		case 'single'
			b = uint8(2);
		case 'int8'
			b = uint8(3);
		case 'uint8'
			b = uint8(4);
		case 'int16'
			b = uint8(5);
		case 'uint16'
			b = uint8(6);
		case 'int32'
			b = uint8(7);
		case 'uint32'
			b = uint8(8);
		case 'int64'
			b = uint8(9);
		case 'uint64'
			b = uint8(10);
		otherwise
			error('Unknown class');
    end
end
